simulink model "torch_pos_with_sensors_tuning(1)"  (R2024a)
settings: Solver=FixedStepAuto  StartTime=0.0  StopTime=50  FixedStep=framePeriod_s  RelTol=1e-3
undefined symbols (not defined in the file): Aircraft, DiscIntNeverNeededParam, framePeriod_s, frameRate_hz, magnitude
libraries: simulink x37, slpidlib x10, simulink_extras x2, dspmathops x1
(part 1 of 4)
settings Model: Creator=brian  LastModifiedBy=lucal
settings SolverCC: AlgebraicLoopSolver=TrustRegion
settings OptimizationCC: DefaultParameterBehavior=Inlined  GainParamInheritBuiltInType=on  UseFloatMulNetSlope=on  DefaultUnderspecifiedDataType=single  EnhancedBackFolding=on  BooleansAsBitfields=on  PassReuseOutputArgsAs=Individual arguments  StateBitsets=on  DataBitsets=on  ActiveStateOutputEnumStorageType=uint16  ZeroExternalMemoryAtStartup=off  ZeroInternalMemoryAtStartup=off  EfficientFloat2IntCast=on  LifeSpan=inf  DifferentSizesBufferReuse=on  OptimizationPriority=RAM  OptimizationCustomize=off  EfficientTunableParamExpr=on
settings DebuggingCC: ParameterPrecisionLossMsg=none  ParameterTunabilityLossMsg=error  UnconnectedInputMsg=warning  UnconnectedOutputMsg=warning  UnconnectedLineMsg=warning  BusObjectLabelMismatch=error  RootOutportRequireBusObject=error  NonBusSignalsTreatedAsBus=error  SFInvalidInputDataAccessInChartInitDiag=error  SFTransitionOutsideNaturalParentDiag=error  SFUnreachableExecutionPathDiag=error  SFUndirectedBroadcastEventsDiag=error
settings HardwareCC: ProdBitPerPointer=32  ProdBitPerSizeT=32  ProdBitPerPtrDiffT=32  ProdLargestAtomicInteger=Long  ProdLargestAtomicFloat=Double  ProdWordSize=32  ProdHWDeviceType=NXP->Cortex-M4  TargetLargestAtomicInteger=Long  TargetLargestAtomicFloat=Double  TargetLongLongMode=on  TargetIntDivRoundTo=Zero  TargetEndianess=LittleEndian  TargetHWDeviceType=NXP->Cortex-M4  ProdEqTarget=off
settings ModelReferenceCC: EnableRefExpFcnMdlSchedulingChecks=on  ModelReferenceNumInstancesAllowed=Single
settings SFSimCC: SimParseCustomCode=off  SimGenImportedTypeDefs=on  MATLABDynamicMemAlloc=off  SimTargetLang=C++
settings SFSimCC: SimUserIncludeDirs=|
  | ../../flight_code/include
  | ../../../ua_spaaro_extra/imu/include
  | ../../../ua_spaaro_extra/gnss/include
  | ../../../ua_spaaro_extra/pres/include
  | ../../../ua_spaaro_extra/sbus/include
  | ../../../ua_spaaro_extra/global_defs/include
settings SFSimCC: SimUserDefines=|
  | SIL
  | __FMU_R_MINI_V1__
settings RTWCC: Description=Embedded Coder  SystemTargetFile=ert.tlc  GenCodeOnly=on  TemplateMakefile=ert_default_tmf  GenerateReport=on  RTWVerbose=off  RTWUseSimCustomCode=on  Toolchain=MinGW64 | gmake (64-bit Windows)  BuildConfiguration=Specify  IncludeHyperlinkInReport=on  LaunchReport=on  TargetLang=C++  GenerateTraceInfo=on  GenerateTraceReport=on  GenerateTraceReportSl=on  GenerateTraceReportSf=on  GenerateTraceReportEml=on  GenerateCodeReplacementReport=on  GPUComputeCapability=3.5  DLArmComputeVersion=19.05
settings RTWCC: CustomInclude=|
  | ../../flight_code/include
  | ../../../ua_spaaro_extra/imu/include
  | ../../../ua_spaaro_extra/gnss/include
  | ../../../ua_spaaro_extra/pres/include
  | ../../../ua_spaaro_extra/sbus/include
  | ../../../ua_spaaro_extra/global_defs/include
settings RTWCC: CustomDefine=|
  | SIL
  | __FMU_R_MINI_V1__
settings CodeAppCC: ForceParamTrailComments=on  IgnoreCustomStorageClasses=off  OperatorAnnotations=on  SimulinkDataObjDesc=on  SFDataObjDesc=on  MATLABFcnDesc=on  CustomSymbolStrGlobalVar=rt$N$M  CustomSymbolStrType=$N$M  CustomSymbolStrFcn=$N$M$F  CustomSymbolStrMacro=$N$M  InsertBlockDesc=on  StateflowObjectComments=on  MATLABSourceComments=on  EnableCustomComments=on  InternalIdentifier=Classic  InlinedPrmAccess=Macros  ReqsInCode=on
settings ERTTargetCC: TargetLangStandard=C++03 (ISO)  GenerateFullHeader=off  IncludeMdlTerminateFcn=off  CombineSignalStateStructs=on  SuppressErrorStatus=on  SupportAbsoluteTime=off  CodeInterfacePackaging=C++ class  SupportNonFinite=off  SupportComplex=off  ParenthesesLevel=Standards  CastingMode=Standards  ERTHeaderFileRootName=autocode$E  ERTSourceFileRootName=autocode$E  InlinedParameterPlacement=NonHierarchical  RootIOFormat=Structure reference  ERTCustomFileTemplate=example_file_process.tlc  ERTFilePackagingFormat=Compact  PreserveExpressionOrder=on  PreserveIfCondition=on  ConvertIfToSwitch=off  EnableSignedLeftShifts=off  EnableSignedRightShifts=off  IndentSize=4

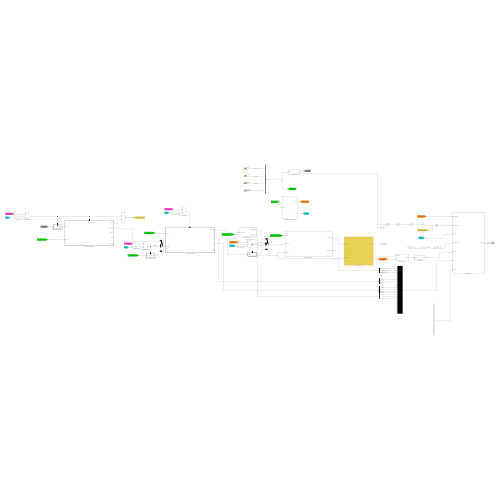
[thumbnail: Simulink's stored preview of the top-level diagram]
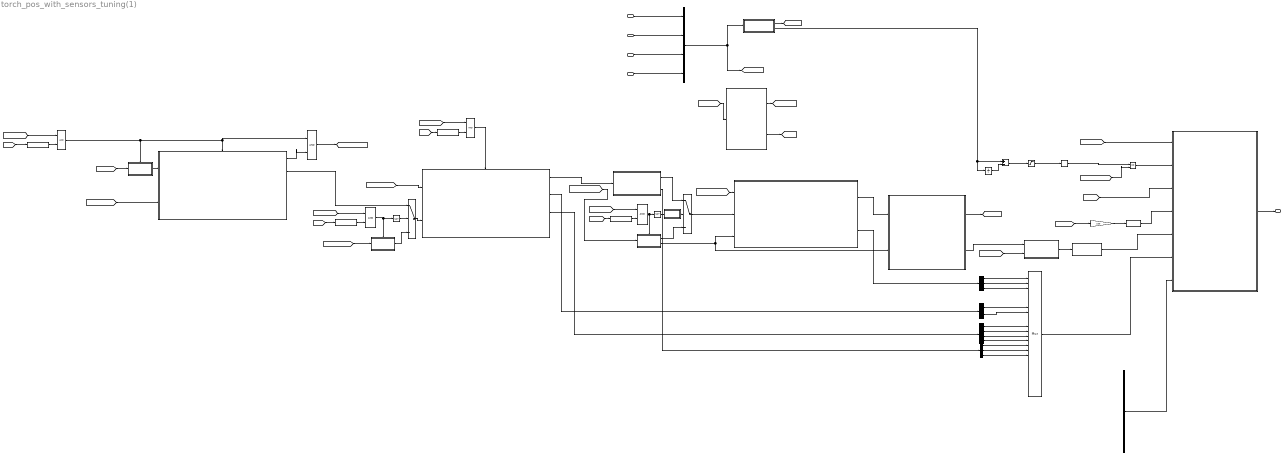
== system torch_pos_with_sensors_tuning(1) ==
  System Data : Inport  OutDataTypeStr=Bus: SysData  SampleTime=framePeriod_s  BusOutputAsStruct=on
  Sensor Data : Inport  Port=2  OutDataTypeStr=Bus: SensorData  SampleTime=framePeriod_s  BusOutputAsStruct=on
  StateEstData : Inport  Port=3  OutDataTypeStr=Bus: StateEstData  SampleTime=framePeriod_s  BusOutputAsStruct=on
  Telemetry Data : Inport  Port=4  OutDataTypeStr=Bus: TelemData  SampleTime=framePeriod_s  BusOutputAsStruct=on
  AND : Logic  IconShape=distinctive  AllPortsSameDT=off  OutDataTypeStr=boolean
  ANGLE CONTROLLER1 : Subsystem
  Bus Creator1 : BusCreator  Inputs=4
  Bus Selector : BusSelector  OutputSignals=throttle,pitch_rate_cmd,pitch_angle_cmd_rad
  Bus Selector1 : BusSelector  OutputSignals=ve_x_cmd,ve_x
  Bus Selector2 : BusSelector  OutputSignals=vz_cmd,vz,tar_z,cur_z
  Cast : DataTypeConversion  OutDataTypeStr=single  SaturateOnIntegerOverflow=off  RndMeth=Floor
  Compare To Constant : simulink/Logic and Bit Operations/Compare To Constant  relop=>  const=0.5  OutDataTypeStr=boolean
  Demux : Demux  Outputs=3
  Gain : Gain  Gain=100
  Motor Mixing Algorithm : Subsystem
  Mux : Mux  Inputs=24
  Mux1 : Mux  Inputs=16
  NOT : Logic  Operator=NOT  IconShape=distinctive  AllPortsSameDT=off  OutDataTypeStr=boolean
  NOT1 : Logic  Operator=NOT  IconShape=distinctive  AllPortsSameDT=off  OutDataTypeStr=boolean
  OR : Logic  Operator=OR  IconShape=distinctive  AllPortsSameDT=off  OutDataTypeStr=boolean
  OUTER_TO_INNER_CONV : Subsystem
  POS_HOLD CONTROLLER : Subsystem
  POS_HOLD_input_conversion : Subsystem
  Saturation : Saturate  UpperLimit=1  LowerLimit=0
  Stab_input_conversion : Subsystem
  Subtract : Sum  Inputs=+-
  Switch : Switch  Criteria=u2 > Threshold  Threshold=0.5  SaturateOnIntegerOverflow=off  InputSameDT=off
  Switch1 : Switch  Criteria=u2 > Threshold  Threshold=0.5  SaturateOnIntegerOverflow=off  InputSameDT=off
  To VMS Data : Subsystem
  Unit Delay : UnitDelay  SampleTime=-1  HasFrameUpgradeWarning=on
  WAYPOINT CONTROLLER : Subsystem
  WAYPOINT CONTROLLER CMD : Subsystem
  cmd to raw pwm1 : Subsystem
  command selection : Subsystem
  compare_to_pos_hold : simulink/Logic and Bit Operations/Compare To Constant  relop=>=  const=2  OutDataTypeStr=boolean
  compare_to_stab : simulink/Logic and Bit Operations/Compare To Constant  relop===  const=1  OutDataTypeStr=boolean
  compare_to_stab1 : simulink/Logic and Bit Operations/Compare To Constant  relop===  const=2  OutDataTypeStr=boolean
  compare_to_wp : simulink/Logic and Bit Operations/Compare To Constant  relop=>=  const=3  OutDataTypeStr=boolean
  delayed : Subsystem
  determine arm and mode selection : Subsystem
  emergency_stop_system1 : Subsystem
  motor_armed AND mode 2 : Logic  IconShape=distinctive  AllPortsSameDT=off  OutDataTypeStr=boolean
  motor_armed AND mode_0 : Logic  IconShape=distinctive  AllPortsSameDT=off  OutDataTypeStr=boolean
  motor_armed AND mode_1 : Logic  IconShape=distinctive  AllPortsSameDT=off  OutDataTypeStr=boolean
  motor_armed AND mode_2 : Logic  IconShape=distinctive  AllPortsSameDT=off  OutDataTypeStr=boolean
  VmsData : Outport  OutDataTypeStr=Bus: VmsData  SampleTime=framePeriod_s  BusOutputAsStruct=on
  wires:
  To VMS Data/1(VmsData) -> VmsData/1  "VmsData"
  [Mode] -> To VMS Data/3(Mode in)
  [arm_state] -> To VMS Data/1(motors_enabled)
  Cast/1 -> To VMS Data/4(throttle_cmd_prcnt)
  [throttle] -> Gain/1
  Gain/1 -> Cast/1
  command selection/1(cmd) -> [cmd]
  Bus Creator1/1 -> command selection/1(InBus), [sys_input]
  [sys_input] -> determine arm and mode selection/1(sys_input)
  Motor Mixing Algorithm/2(PWM) -> emergency_stop_system1/1(input_signal)
  cmd to raw pwm1/1(PwmCmd) -> To VMS Data/5(PWM In)  "PwmCmd"
  emergency_stop_system1/1(pwm_cmd) -> cmd to raw pwm1/1(pwm_cmd)
  Mux/1 -> To VMS Data/6(Aux)
  [arm_state] -> emergency_stop_system1/2(arm)
  compare_to_stab/1 -> motor_armed AND mode_0/2
  [sys_input] -> ANGLE CONTROLLER1/1(Sys_input)
  [arm_state] -> motor_armed AND mode_0/1
  motor_armed AND mode_0/1 -> Stab_input_conversion/Enable, NOT/1
  Stab_input_conversion/1(angle_ctrl_input) -> Switch/3
  [Mode] -> compare_to_stab/1
  ANGLE CONTROLLER1/1(Command out) -> Motor Mixing Algorithm/1(MMA Bus)
  compare_to_pos_hold/1 -> motor_armed AND mode_1/2
  motor_armed AND mode 2/1 -> NOT1/1, POS_HOLD_input_conversion/Enable
  [Mode] -> compare_to_pos_hold/1
  [arm_state] -> motor_armed AND mode_1/1
  NOT1/1 -> Switch1/2
  [arm_state] -> motor_armed AND mode 2/1
  [Mode] -> compare_to_stab1/1
  motor_armed AND mode_1/1 -> POS_HOLD CONTROLLER/Enable
  compare_to_stab1/1 -> motor_armed AND mode 2/2
  Stab_input_conversion/2(low_throttle) -> ANGLE CONTROLLER1/3(low_thottle), Motor Mixing Algorithm/2(low_throttle_flag)
  System Data/1 -> Bus Creator1/1  "Sys Data"
  Sensor Data/1 -> Bus Creator1/2  "Sensor Data"
  StateEstData/1 -> Bus Creator1/3  "StateEstData"
  [sys_input] -> POS_HOLD CONTROLLER/1(Sys_input)
  AND/1 -> [waypoint_reached]
  motor_armed AND mode_2/1 -> WAYPOINT CONTROLLER CMD/Enable, WAYPOINT CONTROLLER/Enable, AND/1
  [arm_state] -> motor_armed AND mode_2/1
  [Mode] -> compare_to_wp/1
  compare_to_wp/1 -> motor_armed AND mode_2/2
  [cmd] -> WAYPOINT CONTROLLER CMD/1(cmd)
  POS_HOLD_input_conversion/1(angle_ctrl_input) -> Switch1/3
  Switch1/1 -> POS_HOLD CONTROLLER/2(param_input)
  POS_HOLD CONTROLLER/2(Output) -> Bus Selector1/1
  WAYPOINT CONTROLLER CMD/1(angle_ctrl_input) -> WAYPOINT CONTROLLER/1(cmd)
  [sys_input] -> WAYPOINT CONTROLLER/2(Sys_input)
  WAYPOINT CONTROLLER/1(wp_reached) -> AND/2
  Mux1/1 -> To VMS Data/7(SBUS in)
  ANGLE CONTROLLER1/2(stab_mode_dbg) -> Bus Selector/1
  Bus Selector/1 -> Mux/1  "<throttle>"
  Bus Selector/2 -> Mux/2  "<pitch_rate_cmd>"
  Bus Selector/3 -> Mux/3  "<pitch_angle_cmd_rad>"
  Bus Selector1/1 -> Mux/7  "<ve_x_cmd>"
  Bus Selector1/2 -> Mux/8  "<ve_x>"
  command selection/2(skip_wp) -> Unit Delay/1, Subtract/1
  Unit Delay/1 -> Subtract/2
  Subtract/1 -> Saturation/1
  Saturation/1 -> Compare To Constant/1
  Telemetry Data/1 -> Bus Creator1/4  "Telemetry Data"
  [sys_input] -> Stab_input_conversion/1(sys_input)
  Switch/1 -> ANGLE CONTROLLER1/2(Param_input)
  Motor Mixing Algorithm/1(throttle) -> [throttle]
  delayed/1(delayed_sig) -> Switch/2
  NOT/1 -> delayed/1(sig)
  POS_HOLD CONTROLLER/1(Command out) -> OUTER_TO_INNER_CONV/1(Outer loop command)
  OUTER_TO_INNER_CONV/1(Inner loop command) -> Switch/1
  WAYPOINT CONTROLLER/2(wp_command) -> Switch1/1
  [sys_input] -> POS_HOLD_input_conversion/1(Sys)
  OR/1 -> To VMS Data/2(waypoint_reached)
  Compare To Constant/1 -> OR/1
  [waypoint_reached] -> OR/2
  POS_HOLD CONTROLLER/3(Output1) -> Bus Selector2/1
  Bus Selector2/1 -> Mux/11  "<vz_cmd>"
  Bus Selector2/2 -> Mux/12  "<vz>"
  Bus Selector2/3 -> Mux/13  "<tar_z>"
  Bus Selector2/4 -> Mux/14  "<cur_z>"
  OUTER_TO_INNER_CONV/2(thrust_vector_cmd) -> Demux/1
  Demux/3 -> Mux/17
  Demux/2 -> Mux/16
  Demux/1 -> Mux/15
  determine arm and mode selection/1(arm_state) -> [arm_state]
  determine arm and mode selection/2(mode) -> [Mode]

== system torch_pos_with_sensors_tuning(1)/ANGLE CONTROLLER1 ==
  Sys_input : Inport
  Param_input : Inport  Port=2
  low_thottle : Inport  Port=3
  Bus Creator : BusCreator  Inputs=3
  Bus Creator4 : BusCreator  Inputs=4
  Bus Selector : BusSelector  OutputSignals=throttle_cc,pitch_angle_cmd_rad
  Ground : Ground
  Ground2 : Ground
  Pitch Controller : Subsystem
  Command out : Outport
  stab_mode_dbg : Outport  Port=2
  wires:
  Bus Creator4/1 -> Command out/1
  Param_input/1 -> Bus Selector/1
  Ground2/1 -> Bus Creator4/4  "yaw_cc"
  Pitch Controller/1(pitch_cc) -> Bus Creator4/3  "pitch_cc"
  Ground/1 -> Bus Creator4/2  "roll_cc"
  Sys_input/1 -> Pitch Controller/1(sys_input)
  Bus Selector/1 -> [throttle_cc]  "<throttle_cc>"
  Bus Selector/2 -> [pitch_angle_cmd_rad]  "<pitch_angle_cmd_rad>"
  [throttle_cc] -> Bus Creator/1, Bus Creator4/1  "throttle"
  [pitch_angle_cmd_rad] -> Pitch Controller/2(Pitch_angle_cmd)
  low_thottle/1 -> [low_throttle_flag]
  [low_throttle_flag] -> Pitch Controller/3(low_throttle_flag)
  Bus Creator/1 -> stab_mode_dbg/1
  [pitch_angle_cmd_rad] -> Bus Creator/3
  Pitch Controller/2(pitch_rate_cmd) -> Bus Creator/2

== system torch_pos_with_sensors_tuning(1)/Motor Mixing Algorithm ==
  MMA Bus : Inport
  low_throttle_flag : Inport  Port=2
  Bus Selector : BusSelector  OutputSignals=throttle,roll_cc,pitch_cc,yaw_cc
  Constant : Constant  OutDataTypeStr=single
  Constant1 : Constant  Value=Aircraft.Control.motor_spin_min  OutDataTypeStr=single
  Constant2 : Constant  Value=[0 0 0 0 0 0 0 0]  OutDataTypeStr=single
  Motor Mix : Constant  Value=Aircraft.Motor.mix  OutDataTypeStr=single
  Multiply : Product  Inputs=**  Multiplication=Matrix(*)  OutDataTypeStr=single
  Mux : Mux
  Reshape : Reshape  OutputDimensionality=Row vector (2-D)
  Saturation Dynamic : simulink/Discontinuities/Saturation Dynamic  OutMin=[]  OutMax=[]  OutDataTypeStr=Inherit: Same as second input  OutDataType=fixdt(1, 16)  OutScaling=2^-10  DoSatur=off
  Switch : Switch  Criteria=u2 > Threshold  SaturateOnIntegerOverflow=off  InputSameDT=off
  Transpose : Math  Operator=transpose
  throttle : Outport
  PWM : Outport  Port=2
  wires:
  Mux/1 -> Reshape/1
  Reshape/1 -> Multiply/1
  Motor Mix/1 -> Transpose/1
  MMA Bus/1 -> Bus Selector/1
  Bus Selector/1 -> Mux/1, throttle/1  "<throttle>"
  Transpose/1 -> Multiply/2
  Saturation Dynamic/1 -> PWM/1
  Constant/1 -> Saturation Dynamic/1
  Constant1/1 -> Saturation Dynamic/3
  Bus Selector/2 -> Mux/2  "<roll_cc>"
  Bus Selector/3 -> Mux/3  "<pitch_cc>"
  Bus Selector/4 -> Mux/4  "<yaw_cc>"
  Switch/1 -> Saturation Dynamic/2
  low_throttle_flag/1 -> Switch/2
  Multiply/1 -> Switch/3  "Command"
  Constant2/1 -> Switch/1

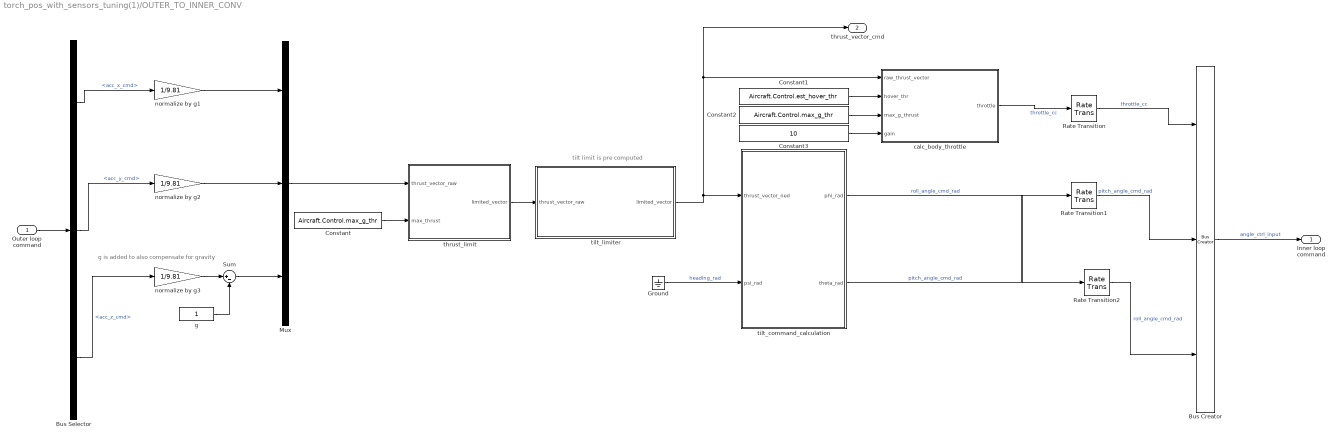
== system torch_pos_with_sensors_tuning(1)/OUTER_TO_INNER_CONV ==
  note: g is added to also compensate for gravity
  note: tilt limit is pre computed
  Outer loop command : Inport
  " tilt_limiter" : MATLAB Function  TreatAsAtomicUnit=on
  Bus Creator : BusCreator  Inputs=3
  Bus Selector : BusSelector  OutputSignals=acc_x_cmd,acc_y_cmd,acc_z_cmd
  Constant : Constant  Value=Aircraft.Control.max_g_thr  OutDataTypeStr=single
  Constant1 : Constant  Value=Aircraft.Control.est_hover_thr  OutDataTypeStr=single
  Constant2 : Constant  Value=Aircraft.Control.max_g_thr  OutDataTypeStr=single
  Constant3 : Constant  Value=10  OutDataTypeStr=single
  Ground : Ground
  Mux : Mux  Inputs=3
  Rate Transition : RateTransition  OutPortSampleTime=0.01
  Rate Transition1 : RateTransition  OutPortSampleTime=0.01
  Rate Transition2 : RateTransition  OutPortSampleTime=0.01
  Sum : Sum  Inputs=|+-
  calc_body_throttle : MATLAB Function  TreatAsAtomicUnit=on
  g : Constant  OutDataTypeStr=single
  normalize by g1 : Gain  Gain=1/9.81
  normalize by g2 : Gain  Gain=1/9.81
  normalize by g3 : Gain  Gain=1/9.81
  thrust_limit : MATLAB Function  TreatAsAtomicUnit=on
  tilt_command_calculation : MATLAB Function  TreatAsAtomicUnit=on
  Inner loop command : Outport
  thrust_vector_cmd : Outport  Port=2
  wires:
  Constant/1 -> thrust_limit/2(max_thrust)
  Mux/1 -> thrust_limit/1(thrust_vector_raw)
  Outer loop command/1 -> Bus Selector/1
  Bus Selector/1 -> normalize by g1/1  "<acc_x_cmd>"
  Bus Selector/2 -> normalize by g2/1  "<acc_y_cmd>"
  Bus Creator/1 -> Inner loop command/1  "angle_ctrl_input"
  Ground/1 -> tilt_command_calculation/2(psi_rad)  "heading_rad"
  Bus Selector/3 -> normalize by g3/1  "<acc_z_cmd>"
  g/1 -> Sum/2
  normalize by g3/1 -> Sum/1
  normalize by g1/1 -> Mux/1
  normalize by g2/1 -> Mux/2
  Sum/1 -> Mux/3
  thrust_limit/1(limited_vector) -> " tilt_limiter"/1(thrust_vector_raw)
  tilt_command_calculation/1(phi_rad) -> Rate Transition2/1  "roll_angle_cmd_rad"
  tilt_command_calculation/2(theta_rad) -> Rate Transition1/1  "pitch_angle_cmd_rad"
  calc_body_throttle/1(throttle) -> Rate Transition/1  "throttle_cc"
  " tilt_limiter"/1(limited_vector) -> tilt_command_calculation/1(thrust_vector_ned), thrust_vector_cmd/1, calc_body_throttle/1(raw_thrust_vector)
  Constant1/1 -> calc_body_throttle/2(hover_thr)
  Constant2/1 -> calc_body_throttle/3(max_g_thrust)
  Constant3/1 -> calc_body_throttle/4(gain)
  Rate Transition/1 -> Bus Creator/1  "throttle_cc"
  Rate Transition1/1 -> Bus Creator/2  "pitch_angle_cmd_rad"
  Rate Transition2/1 -> Bus Creator/3  "roll_angle_cmd_rad"

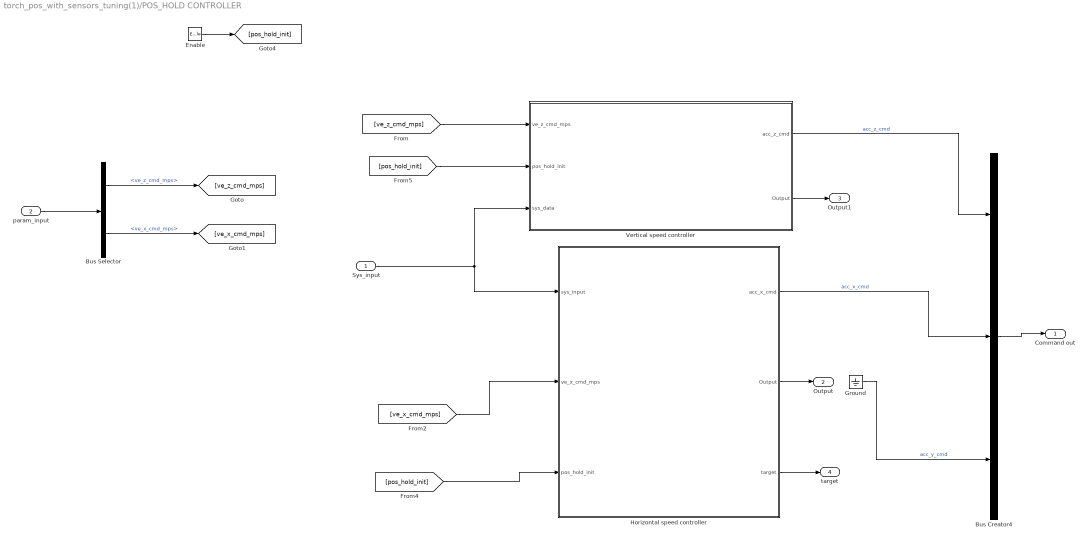
== system torch_pos_with_sensors_tuning(1)/POS_HOLD CONTROLLER ==
  Sys_input : Inport
  param_input : Inport  Port=2
  Enable : EnablePort  StatesWhenEnabling=reset  PropagateVarSize=During execution  ShowOutputPort=on
  Bus Creator4 : BusCreator  Inputs=3
  Bus Selector : BusSelector  OutputSignals=ve_z_cmd_mps,ve_x_cmd_mps
  Ground : Ground
  Horizontal speed controller : Subsystem
  Vertical speed controller : Subsystem
  Command out : Outport
  Output : Outport  Port=2
  Output1 : Outport  Port=3
  target : Outport  Port=4
  wires:
  Bus Creator4/1 -> Command out/1
  Bus Selector/1 -> [ve_z_cmd_mps]  "<ve_z_cmd_mps>"
  Bus Selector/2 -> [ve_x_cmd_mps]  "<ve_x_cmd_mps>"
  param_input/1 -> Bus Selector/1
  Enable/1 -> [pos_hold_init]
  Vertical speed controller/1(acc_z_cmd) -> Bus Creator4/1  "acc_z_cmd"
  Horizontal speed controller/1(acc_x_cmd) -> Bus Creator4/2  "acc_x_cmd"
  Ground/1 -> Bus Creator4/3  "acc_y_cmd"
  [ve_x_cmd_mps] -> Horizontal speed controller/2(ve_x_cmd_mps)
  Sys_input/1 -> Vertical speed controller/3(sys_data), Horizontal speed controller/1(sys_input)
  [pos_hold_init] -> Horizontal speed controller/3(pos_hold_init)
  Horizontal speed controller/2(Output) -> Output/1
  [ve_z_cmd_mps] -> Vertical speed controller/1(ve_z_cmd_mps)
  [pos_hold_init] -> Vertical speed controller/2(pos_hold_init)
  Vertical speed controller/2(Output) -> Output1/1
  Horizontal speed controller/3(target) -> target/1

== system torch_pos_with_sensors_tuning(1)/POS_HOLD_input_conversion ==
  Sys : Inport
  Enable : EnablePort
  Bus Creator : BusCreator  Inputs=4
  Bus Selector2 : BusSelector  OutputSignals=Telemetry Data.param
  Cast1 : DataTypeConversion  OutDataTypeStr=single  SaturateOnIntegerOverflow=off  RndMeth=Floor
  Cast2 : DataTypeConversion  OutDataTypeStr=single  SaturateOnIntegerOverflow=off  RndMeth=Floor
  Constant3 : Constant  Value=-0.5
  Constant4 : Constant  Value=0.5
  Constant5 : Constant  Value=-0.5
  Constant6 : Constant  Value=0.5
  Ground : Ground
  Ground2 : Ground
  Saturation Dynamic : simulink/Discontinuities/Saturation Dynamic  OutMin=[]  OutMax=[]  OutDataTypeStr=double  OutDataType=fixdt(1, 16)  OutScaling=2^-10  DoSatur=off
  Saturation Dynamic1 : simulink/Discontinuities/Saturation Dynamic  OutMin=[]  OutMax=[]  OutDataTypeStr=double  OutDataType=fixdt(1, 16)  OutScaling=2^-10  DoSatur=off
  Selector : Selector  IndexMode=Zero-based  InputPortWidth=24  IndexOptions=Index vector (dialog)  Indices=1  OutputSizes=1
  Selector1 : Selector  IndexMode=Zero-based  InputPortWidth=24  IndexOptions=Index vector (dialog)  Indices=2  OutputSizes=1
  angle_ctrl_input : Outport
  wires:
  Bus Creator/1 -> angle_ctrl_input/1  "pos_hold_cmd"
  Saturation Dynamic/1 -> Bus Creator/1  "ve_z_cmd_mps"
  Saturation Dynamic1/1 -> Bus Creator/2  "ve_x_cmd_mps"
  Ground2/1 -> Bus Creator/3  "ve_y_cmd_mps"
  Sys/1 -> Bus Selector2/1
  Constant5/1 -> Saturation Dynamic/3
  Constant6/1 -> Saturation Dynamic/1
  Cast1/1 -> Saturation Dynamic/2
  Selector/1 -> Cast1/1
  Bus Selector2/1 -> Selector1/1, Selector/1  "<param>"
  Ground/1 -> Bus Creator/4  "yaw_rate_cmd_radps"
  Constant4/1 -> Saturation Dynamic1/1
  Constant3/1 -> Saturation Dynamic1/3
  Cast2/1 -> Saturation Dynamic1/2
  Selector1/1 -> Cast2/1

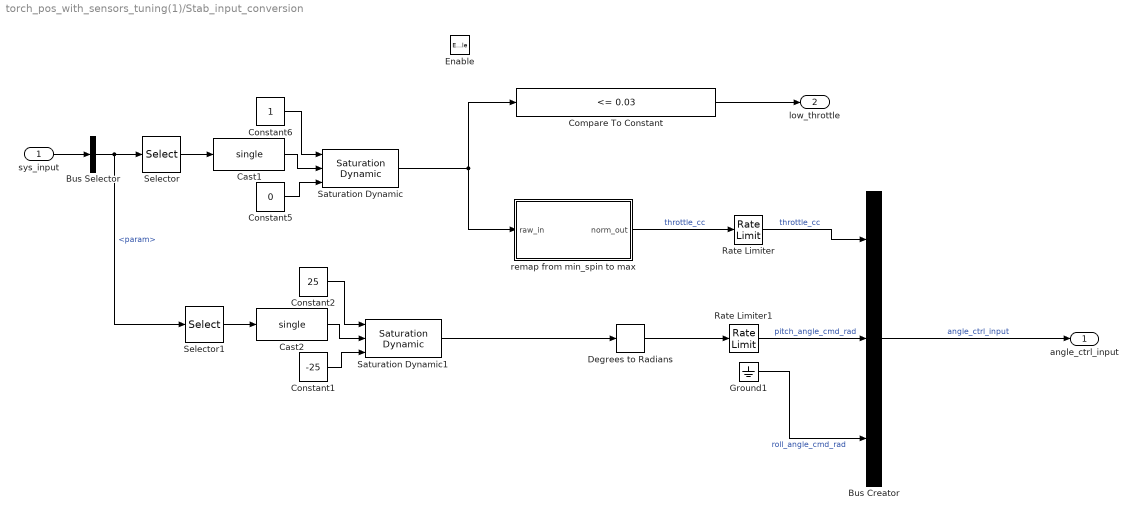
== system torch_pos_with_sensors_tuning(1)/Stab_input_conversion ==
  sys_input : Inport
  Enable : EnablePort
  Bus Creator : BusCreator  Inputs=3
  Bus Selector : BusSelector  OutputSignals=Telemetry Data.param
  Cast1 : DataTypeConversion  OutDataTypeStr=single  SaturateOnIntegerOverflow=off  RndMeth=Floor
  Cast2 : DataTypeConversion  OutDataTypeStr=single  SaturateOnIntegerOverflow=off  RndMeth=Floor
  Compare To Constant : simulink/Logic and Bit Operations/Compare To Constant  relop=<=  const=0.03  OutDataTypeStr=boolean
  Constant1 : Constant  Value=-25
  Constant2 : Constant  Value=25
  Constant5 : Constant  Value=0
  Constant6 : Constant
  Degrees to Radians : simulink_extras/Transformations/Degrees to Radians
  Ground1 : Ground
  Rate Limiter : RateLimiter  SampleTimeMode=inherited
  Rate Limiter1 : RateLimiter  RisingSlewLimit=2  SampleTimeMode=inherited
  Saturation Dynamic : simulink/Discontinuities/Saturation Dynamic  OutMin=[]  OutMax=[]  OutDataTypeStr=double  OutDataType=fixdt(1, 16)  OutScaling=2^-10  DoSatur=off
  Saturation Dynamic1 : simulink/Discontinuities/Saturation Dynamic  OutMin=[]  OutMax=[]  OutDataTypeStr=double  OutDataType=fixdt(1, 16)  OutScaling=2^-10  DoSatur=off
  Selector : Selector  IndexMode=Zero-based  InputPortWidth=24  IndexOptions=Index vector (dialog)  Indices=1  OutputSizes=1
  Selector1 : Selector  IndexMode=Zero-based  InputPortWidth=24  IndexOptions=Index vector (dialog)  Indices=2  OutputSizes=1
  remap from min_spin to max : Subsystem
  angle_ctrl_input : Outport
  low_throttle : Outport  Port=2
  wires:
  Ground1/1 -> Bus Creator/3  "roll_angle_cmd_rad"
  remap from min_spin to max/1(norm_out) -> Rate Limiter/1  "throttle_cc"
  Bus Creator/1 -> angle_ctrl_input/1  "angle_ctrl_input"
  Saturation Dynamic1/1 -> Degrees to Radians/1
  sys_input/1 -> Bus Selector/1
  Constant5/1 -> Saturation Dynamic/3
  Constant6/1 -> Saturation Dynamic/1
  Bus Selector/1 -> Selector1/1, Selector/1  "<param>"
  Selector/1 -> Cast1/1
  Cast1/1 -> Saturation Dynamic/2
  Compare To Constant/1 -> low_throttle/1
  Saturation Dynamic/1 -> Compare To Constant/1, remap from min_spin to max/1(raw_in)
  Rate Limiter/1 -> Bus Creator/1  "throttle_cc"
  Constant1/1 -> Saturation Dynamic1/3
  Selector1/1 -> Cast2/1
  Cast2/1 -> Saturation Dynamic1/2
  Constant2/1 -> Saturation Dynamic1/1
  Degrees to Radians/1 -> Rate Limiter1/1
  Rate Limiter1/1 -> Bus Creator/2  "pitch_angle_cmd_rad"

== system torch_pos_with_sensors_tuning(1)/To VMS Data ==
  motors_enabled : Inport
  waypoint_reached : Inport  Port=2
  Mode in : Inport  Port=3
  throttle_cmd_prcnt : Inport  Port=4
  PWM In : Inport  Port=5
  Aux : Inport  Port=6
  SBUS in : Inport  Port=7
  Bus Creator : BusCreator  Inputs=9  OutDataTypeStr=Bus: VmsData  NonVirtualBus=on
      settings: InheritFromInputs=off
  Ground : Ground
  Ground2 : Ground
  VmsData : Outport
  wires:
  Bus Creator/1 -> VmsData/1
  waypoint_reached/1 -> Bus Creator/1  "advance_waypoint"
  motors_enabled/1 -> Bus Creator/2  "motors_enabled"
  Mode in/1 -> Bus Creator/3  "mode"
  SBUS in/1 -> Bus Creator/4  "sbus"
  PWM In/1 -> Bus Creator/5  "pwm"
  throttle_cmd_prcnt/1 -> Bus Creator/6  "throttle_cmd_prcnt"
  Aux/1 -> Bus Creator/9  "aux"
  Ground/1 -> Bus Creator/7  "flight_time_remaining_s"
  Ground2/1 -> Bus Creator/8  "power_remaining_prcnt"

== system torch_pos_with_sensors_tuning(1)/WAYPOINT CONTROLLER ==
  cmd : Inport
  Sys_input : Inport  Port=2
  Enable : EnablePort  StatesWhenEnabling=reset  ShowOutputPort=on
  Bus Selector1 : BusSelector  OutputSignals=Telemetry Data.waypoints_updated,Telemetry Data.current_waypoint
  Constant : Constant  OutDataTypeStr=int16
  OR : Logic  Operator=OR  Inputs=3  IconShape=distinctive  AllPortsSameDT=off  OutDataTypeStr=boolean
  Sum : Sum  Inputs=|++
  Unit Delay : UnitDelay  SampleTime=-1  HasFrameUpgradeWarning=on
  WP_NAV : Subsystem
  capture rising edge : Subsystem
  determine target : Subsystem
  wp_completion_check : Subsystem
  wp_reached : Outport
  wp_command : Outport  Port=2
  tar_pos_m : Outport  Port=3
  cur_wp : Outport  Port=4
  bearing_to_tar : Outport  Port=5
  wires:
  Sys_input/1 -> Bus Selector1/1, WP_NAV/2(Sys_input), wp_completion_check/2(Sys_input), determine target/1(sys_input)
  Enable/1 -> WP_NAV/Enable
  WP_NAV/1(Command out) -> wp_command/1
  determine target/1(cur_target_pos_m) -> wp_completion_check/1(target_pos), tar_pos_m/1, WP_NAV/3(cur_target_pos_m)  "cur_target_pos_m"
  OR/1 -> determine target/Enable  "enable"
  Bus Selector1/1 -> OR/1  "<waypoints_updated>"
  capture rising edge/1(enable) -> OR/2
  Unit Delay/1 -> OR/3
  cmd/1 -> WP_NAV/1(Cmd)
  wp_completion_check/1(wp_reached) -> wp_reached/1, Unit Delay/1
  Constant/1 -> Sum/2
  Bus Selector1/2 -> Sum/1  "<current_waypoint>"
  Sum/1 -> cur_wp/1, capture rising edge/1(<current_waypoint>)  "cur_wp"
  determine target/2(prev_pos_m) -> WP_NAV/4(prev_pos_m)  "prev_wp"
  determine target/3(max_v_xy_mps) -> WP_NAV/5(max_v_hor_mps)
  determine target/4(max_v_z_mps) -> WP_NAV/6(max_v_z_mps)
  WP_NAV/2(nav_data) -> bearing_to_tar/1

== system torch_pos_with_sensors_tuning(1)/WAYPOINT CONTROLLER CMD ==
  cmd : Inport
  Enable : EnablePort
  Bus Creator : BusCreator  Inputs=4
  Bus Selector2 : BusSelector  OutputSignals=throttle,pitch,roll,yaw
  Constant : Constant  Commented=on  Value=Aircraft.Inceptor.deadband
  Constant1 : Constant  Value=Aircraft.Control.v_hor_max  OutDataTypeStr=single
  Constant4 : Constant  Value=Aircraft.Control.v_hor_max  OutDataTypeStr=single
  Ground : Ground
  Product : Product
  Product1 : Product
  Product2 : Product
  Throttle Mapper : Subsystem  Commented=on
  pitch_norm_deadband : Subsystem  Commented=on
  remap from min_spin to max : Subsystem
  angle_ctrl_input : Outport
  wires:
  Bus Selector2/3 -> Product2/1  "<roll>"
  Product2/1 -> Bus Creator/3  "vb_y_cmd_mps"
  Bus Selector2/2 -> Product1/1  "<pitch>"
  Bus Creator/1 -> angle_ctrl_input/1  "angle_ctrl_input"
  Product1/1 -> Bus Creator/2  "vb_x_cmd_mps"
  cmd/1 -> Bus Selector2/1
  Product/1 -> Bus Creator/4  "yaw_rate_cmd_radps"
  Bus Selector2/4 -> Product/1  "<yaw>"
  pitch_norm_deadband/1(normalized_out) -> Throttle Mapper/1(Throttle)
  Constant/1 -> pitch_norm_deadband/2(deadband)
  Constant1/1 -> Product1/2
  Constant4/1 -> Product2/2
  Ground/1 -> Product/2
  remap from min_spin to max/1(norm_out) -> Bus Creator/1  "ve_z_cmd_mps"
  Bus Selector2/1 -> remap from min_spin to max/1(raw_in)  "<throttle>"

== system torch_pos_with_sensors_tuning(1)/cmd to raw pwm1 ==
  note: cnt - pwm output to actual hardware
  pwm_cmd : Inport
  Data Type Conversion : DataTypeConversion  OutDataTypeStr=int16  SaturateOnIntegerOverflow=off  RndMeth=Floor
  motor_PWM_denormalize : Subsystem
  PwmCmd : Outport
  wires:
  pwm_cmd/1 -> motor_PWM_denormalize/1(normalized_input)  "cmd"
  Data Type Conversion/1 -> PwmCmd/1  "cnt"
  motor_PWM_denormalize/1(raw_output) -> Data Type Conversion/1

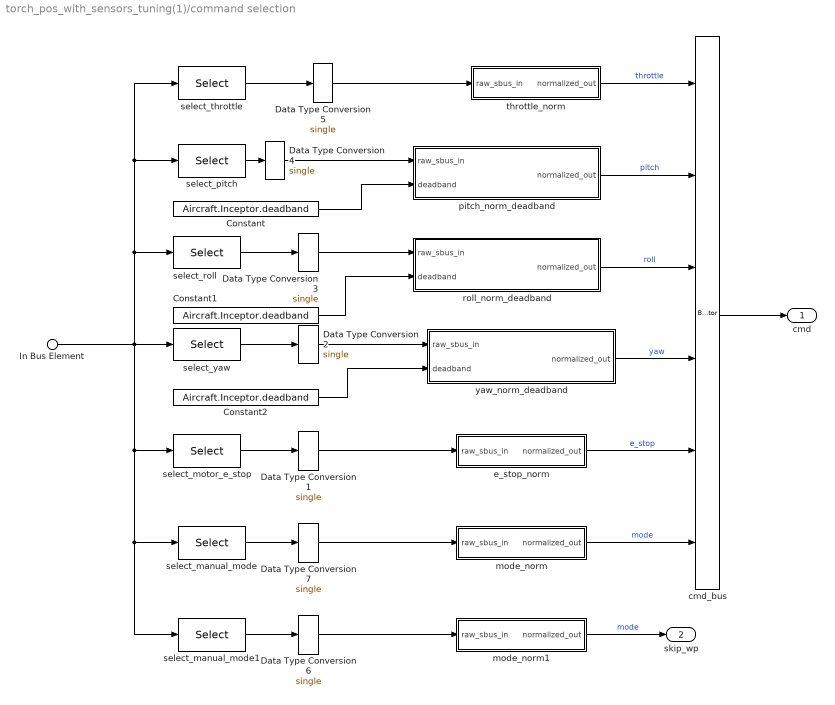
== system torch_pos_with_sensors_tuning(1)/command selection ==
  In Bus Element : Inport  PortName=InBus  Element=Sensor Data.inceptor.ch
  Constant : Constant  Value=Aircraft.Inceptor.deadband  OutDataTypeStr=single
  Constant1 : Constant  Value=Aircraft.Inceptor.deadband  OutDataTypeStr=single
  Constant2 : Constant  Value=Aircraft.Inceptor.deadband  OutDataTypeStr=single
  Data Type Conversion{1..7} (7 alike) : DataTypeConversion  OutDataTypeStr=single  SaturateOnIntegerOverflow=off  RndMeth=Floor
  cmd_bus : BusCreator  Inputs=6
  e_stop_norm : Subsystem
  mode_norm : Subsystem
  mode_norm1 : Subsystem
  pitch_norm_deadband : Subsystem
  roll_norm_deadband : Subsystem
  select_manual_mode : Selector  IndexOptions=Index vector (dialog)  Indices=Aircraft.Inceptor.mode0  OutputSizes=1
  select_manual_mode1 : Selector  IndexOptions=Index vector (dialog)  Indices=9  OutputSizes=1
  select_motor_e_stop : Selector  IndexOptions=Index vector (dialog)  Indices=Aircraft.Inceptor.throttle_e_stop  OutputSizes=1
  select_pitch : Selector  IndexOptions=Index vector (dialog)  Indices=Aircraft.Inceptor.pitch  OutputSizes=1
  select_roll : Selector  IndexOptions=Index vector (dialog)  Indices=Aircraft.Inceptor.roll  OutputSizes=1
  select_throttle : Selector  IndexOptions=Index vector (dialog)  Indices=Aircraft.Inceptor.throttle  OutputSizes=1
  select_yaw : Selector  IndexOptions=Index vector (dialog)  Indices=Aircraft.Inceptor.yaw  OutputSizes=1
  throttle_norm : Subsystem
  yaw_norm_deadband : Subsystem
  cmd : Outport
  skip_wp : Outport  Port=2
  wires:
  select_pitch/1 -> Data Type Conversion4/1
  select_yaw/1 -> Data Type Conversion2/1
  select_throttle/1 -> Data Type Conversion5/1
  cmd_bus/1 -> cmd/1
  Data Type Conversion5/1 -> throttle_norm/1(raw_sbus_in)
  select_roll/1 -> Data Type Conversion3/1
  In Bus Element/1 -> select_roll/1, select_throttle/1, select_pitch/1, select_manual_mode/1, select_manual_mode1/1, select_motor_e_stop/1, select_yaw/1
  Data Type Conversion1/1 -> e_stop_norm/1(raw_sbus_in)
  select_motor_e_stop/1 -> Data Type Conversion1/1
  Data Type Conversion7/1 -> mode_norm/1(raw_sbus_in)
  select_manual_mode/1 -> Data Type Conversion7/1
  Data Type Conversion2/1 -> yaw_norm_deadband/1(raw_sbus_in)
  Constant2/1 -> yaw_norm_deadband/2(deadband)
  throttle_norm/1(normalized_out) -> cmd_bus/1  "throttle"
  roll_norm_deadband/1(normalized_out) -> cmd_bus/3  "roll"
  pitch_norm_deadband/1(normalized_out) -> cmd_bus/2  "pitch"
  Data Type Conversion4/1 -> pitch_norm_deadband/1(raw_sbus_in)
  Constant/1 -> pitch_norm_deadband/2(deadband)
  Constant1/1 -> roll_norm_deadband/2(deadband)
  Data Type Conversion3/1 -> roll_norm_deadband/1(raw_sbus_in)
  yaw_norm_deadband/1(normalized_out) -> cmd_bus/4  "yaw"
  e_stop_norm/1(normalized_out) -> cmd_bus/5  "e_stop"
  mode_norm/1(normalized_out) -> cmd_bus/6  "mode"
  select_manual_mode1/1 -> Data Type Conversion6/1
  Data Type Conversion6/1 -> mode_norm1/1(raw_sbus_in)
  mode_norm1/1(normalized_out) -> skip_wp/1  "mode"

== system torch_pos_with_sensors_tuning(1)/delayed ==
  sig : Inport
  Constant : Constant  Value=framePeriod_s  OutDataTypeStr=single
  Constant1 : Constant  Value=0.5  OutDataTypeStr=single
  Delay : Delay  DelayLengthSource=Input port
      settings: InputPortMap=u0,p1
  Divide : Product  Inputs=*/
  delayed_sig : Outport
  wires:
  Delay/1 -> delayed_sig/1
  sig/1 -> Delay/1
  Divide/1 -> Delay/2
  Constant/1 -> Divide/2
  Constant1/1 -> Divide/1

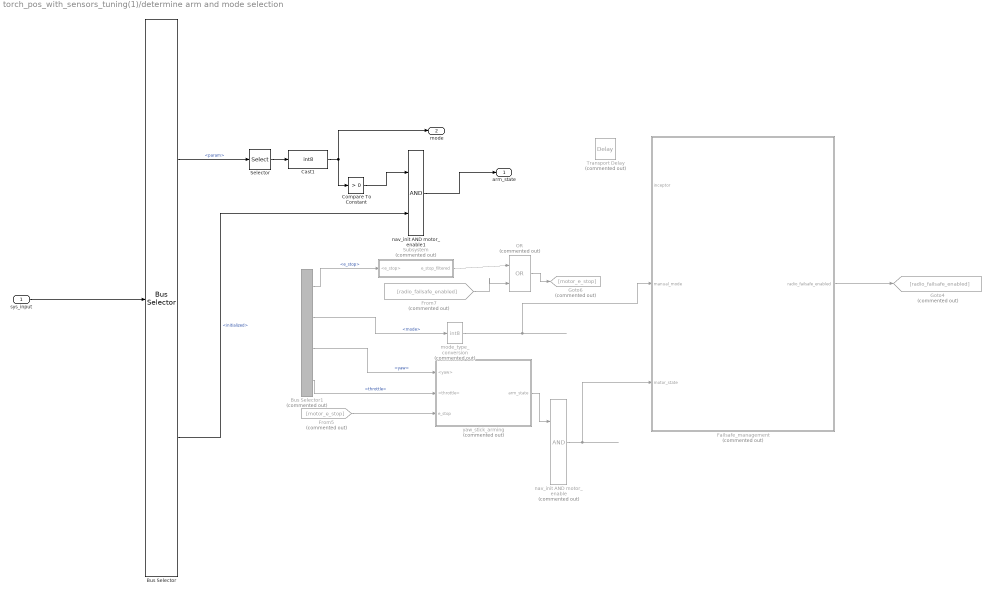
== system torch_pos_with_sensors_tuning(1)/determine arm and mode selection ==
  sys_input : Inport
  Bus Selector : BusSelector  OutputSignals=Telemetry Data.param,StateEstData.bfs_ins.initialized
  Bus Selector1 : BusSelector  Commented=on  OutputSignals=e_stop,mode,yaw,throttle
  Cast1 : DataTypeConversion  OutDataTypeStr=int8  SaturateOnIntegerOverflow=off  RndMeth=Floor
  Compare To Constant : simulink/Logic and Bit Operations/Compare To Constant  relop=>  const=0  OutDataTypeStr=boolean
  Failsafe_management : Subsystem  Commented=on
  From5 : From  Commented=on  GotoTag=motor_e_stop
  From7 : From  Commented=on  GotoTag=radio_failsafe_enabled
  Goto4 : Goto  Commented=on  GotoTag=radio_failsafe_enabled
  Goto6 : Goto  Commented=on  GotoTag=motor_e_stop
  OR : Logic  Commented=on  Operator=OR  IconShape=distinctive  AllPortsSameDT=off  OutDataTypeStr=boolean
  Selector : Selector  IndexMode=Zero-based  InputPortWidth=24  IndexOptions=Index vector (dialog)  Indices=0  OutputSizes=1
  Subsystem : Subsystem  Commented=on
  Transport Delay : TransportDelay  Commented=on
  mode_type_conversion : DataTypeConversion  Commented=on  OutDataTypeStr=int8  RndMeth=Nearest  SaturateOnIntegerOverflow=off
  nav_init AND motor_enable : Logic  Commented=on  IconShape=distinctive  AllPortsSameDT=off  OutDataTypeStr=boolean
  nav_init AND motor_enable1 : Logic  IconShape=distinctive  AllPortsSameDT=off  OutDataTypeStr=boolean
  yaw_stick_arming : Subsystem  Commented=on
  arm_state : Outport
  mode : Outport  Port=2
  wires:
  Selector/1 -> Cast1/1
  Bus Selector/1 -> Selector/1  "<param>"
  Bus Selector1/1 -> Subsystem/1(<e_stop>)  "<e_stop>"
  Cast1/1 -> Compare To Constant/1, mode/1
  OR/1 -> Goto6/1
  Bus Selector/2 -> nav_init AND motor_enable1/2  "<initialized>"
  nav_init AND motor_enable1/1 -> arm_state/1
  Compare To Constant/1 -> nav_init AND motor_enable1/1
  Subsystem/1(e_stop_filtered) -> OR/1
  Bus Selector1/4 -> yaw_stick_arming/2(<throttle>)  "<throttle>"
  From5/1 -> yaw_stick_arming/3(e_stop)
  Bus Selector1/3 -> yaw_stick_arming/1(<yaw>)  "<yaw>"
  yaw_stick_arming/1(arm_state) -> nav_init AND motor_enable/1
  nav_init AND motor_enable/1 -> Failsafe_management/3(motor_state)
  mode_type_conversion/1 -> Failsafe_management/2(manual_mode)
  Bus Selector1/2 -> mode_type_conversion/1  "<mode>"
  sys_input/1 -> Bus Selector/1
  Failsafe_management/1(radio_failsafe_enabled) -> Goto4/1
  From7/1 -> OR/2

== system torch_pos_with_sensors_tuning(1)/emergency_stop_system1 ==
  input_signal : Inport
  arm : Inport  Port=2
  Constant : Constant  Value=[0,0,0,0,0,0,0,0]  OutDataTypeStr=single
  emergency_switch : Switch  Criteria=u2 > Threshold  Threshold=0.5  SaturateOnIntegerOverflow=off  InputSameDT=off
  pwm_cmd : Outport
  wires:
  emergency_switch/1 -> pwm_cmd/1
  arm/1 -> emergency_switch/2
  input_signal/1 -> emergency_switch/1
  Constant/1 -> emergency_switch/3

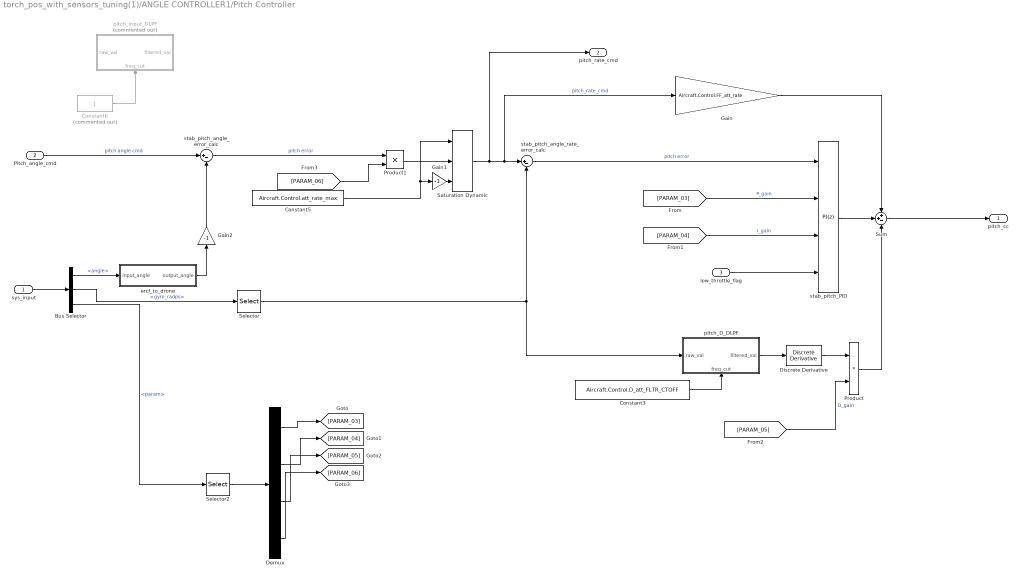
== system torch_pos_with_sensors_tuning(1)/ANGLE CONTROLLER1/Pitch Controller ==
  sys_input : Inport
  Pitch_angle_cmd : Inport  Port=2
  low_throttle_flag : Inport  Port=3
  Bus Selector : BusSelector  OutputSignals=Sensor Data.ercf.angle,StateEstData.bfs_ins.gyro_radps,Telemetry Data.param
  Constant3 : Constant  Value=Aircraft.Control.D_att_FLTR_CTOFF  OutDataTypeStr=single
  Constant5 : Constant  Value=Aircraft.Control.att_rate_max  OutDataTypeStr=single
  Constant6 : Constant  Commented=on  OutDataTypeStr=single
  Demux : Demux
  Discrete Derivative : simulink/Discrete/Discrete Derivative  gainval=1.0  ICPrevScaledInput=0.0  OutMin=[]  OutMax=[]  OutDataType=fixdt(1, 16)  OutScaling=2^-10  DoSatur=off
  Gain : Gain  Gain=Aircraft.Control.FF_att_rate
  Gain1 : Gain  Gain=-1
  Gain2 : Gain  Gain=-1
  Product : Product
  Product1 : Product
  Saturation Dynamic : simulink/Discontinuities/Saturation Dynamic  OutMin=[]  OutMax=[]  OutDataTypeStr=Inherit: Same as second input  OutDataType=fixdt(1, 16)  OutScaling=2^-10  DoSatur=off
  Selector : Selector  IndexMode=Zero-based  InputPortWidth=3  IndexOptions=Index vector (dialog)  Indices=1  OutputSizes=1
  Selector2 : Selector  IndexMode=Zero-based  InputPortWidth=24  IndexOptions=Index vector (dialog)  Indices=[3 4 5 6]  OutputSizes=1
  Sum : Sum  Inputs=++-
  ercf_to_drone : MATLAB Function  TreatAsAtomicUnit=on
  pitch_D_DLPF : Subsystem
      settings: PortSchema="{\"entries\":[{\"content\":{\"sides\":[{\"content\":{\"connectorIds\":[\"In1\"]},\"type\":\"ConnectorPlacement.EquallySpacedRectSide\",\"uuid\":\"20236834-aeb3-4c5b-bb2e-f84447e752b5\"},{\"content\":{\"connectorIds\":[\"Out1\"],\"side\":\"RIGHT\"},\"type\":\"ConnectorPlacement.EquallySpacedRectSide\",\"uuid\":\"d668f9a1-a3df-4207-8bf1-99fb838e59b2\"},{\"content\":{\"connectorIds\":[],\"side\":\"TOP\"},\"type\":\"ConnectorPlacement.EquallySpacedRectSide\",\"uuid\":\"66cceb06-f4bc-4278-b965-2427292e46df\"},{\"content\":{\"connectorIds\":[\"In2\"],\"side\":\"BOTTOM\"},\"type\":\"ConnectorPlacement.EquallySpacedRectSide\",\"uuid\":\"8fdaac6a-cb03-4bd4-87bb-7bafd10bc297\"}]},\"type\":\"ConnectorPlacement.EquallySpacedConnector\",\"uuid\":\"3dc29a9a-e794-478d-b7df-452e6c2d3f66\"}],\"packageUris\":[\"http://schema.mathworks.com/mf0/Connector/R2020b\"],\"version\":\"1.0\"}"
  pitch_input_DLPF : Subsystem  Commented=on
      settings: PortSchema="{\"entries\":[{\"content\":{\"sides\":[{\"content\":{\"connectorIds\":[\"In1\"]},\"type\":\"ConnectorPlacement.EquallySpacedRectSide\",\"uuid\":\"20236834-aeb3-4c5b-bb2e-f84447e752b5\"},{\"content\":{\"connectorIds\":[\"Out1\"],\"side\":\"RIGHT\"},\"type\":\"ConnectorPlacement.EquallySpacedRectSide\",\"uuid\":\"d668f9a1-a3df-4207-8bf1-99fb838e59b2\"},{\"content\":{\"connectorIds\":[],\"side\":\"TOP\"},\"type\":\"ConnectorPlacement.EquallySpacedRectSide\",\"uuid\":\"66cceb06-f4bc-4278-b965-2427292e46df\"},{\"content\":{\"connectorIds\":[\"In2\"],\"side\":\"BOTTOM\"},\"type\":\"ConnectorPlacement.EquallySpacedRectSide\",\"uuid\":\"8fdaac6a-cb03-4bd4-87bb-7bafd10bc297\"}]},\"type\":\"ConnectorPlacement.EquallySpacedConnector\",\"uuid\":\"3dc29a9a-e794-478d-b7df-452e6c2d3f66\"}],\"packageUris\":[\"http://schema.mathworks.com/mf0/Connector/R2020b\"],\"version\":\"1.0\"}"
  stab_pitch_PID : slpidlib/PID Controller  Controller=PI  Form=Parallel  TimeDomain=Discrete-time  UseExternalTs=off  SampleTime=framePeriod_s  IntegratorMethod=Forward Euler  FilterMethod=Forward Euler  ControllerParametersSource=external  P=0.335  I=0.005  UseKiTs=off  D=0  UseExternalDerivativeSource=off  N=100  UseFilter=off  TunerSelectOption=Transfer Function Based (PID Tuner App)  InitialConditionSource=internal  InitialConditionForIntegrator=0  InitialConditionForFilter=0  DifferentiatorICPrevScaledInput=0  ExternalReset=either  TrackingMode=off  Kt=1  LimitOutput=on  SatLimitsSource=internal  UpperSaturationLimit=1  LowerSaturationLimit=-1  LinearizeAsGain=on  AntiWindupMode=clamping  Kb=1  LimitIntegrator=off  UpperIntegratorSaturationLimit=inf  LowerIntegratorSaturationLimit=-inf  POutMin=[]  POutMax=[]  IOutMin=[]  IOutMax=[]  DOutMin=[]  DOutMax=[]  NOutMin=[]  NOutMax=[]  SumOutMin=[]  SumOutMax=[]  SaturationOutMin=[]  SaturationOutMax=[]  PParamMin=[]  PParamMax=[]  IParamMin=[]  IParamMax=[]  DParamMin=[]  DParamMax=[]  NParamMin=[]  NParamMax=[]  KbParamMin=[]  KbParamMax=[]  KtParamMin=[]  KtParamMax=[]  KbOutMin=[]  KbOutMax=[]  KtOutMin=[]  KtOutMax=[]  IntegratorOutMin=[]  IntegratorOutMax=[]  FilterOutMin=[]  FilterOutMax=[]  SumI1OutMin=[]  SumI1OutMax=[]  SumI2OutMin=[]  SumI2OutMax=[]  SumI3OutMin=[]  SumI3OutMax=[]  SumI4OutMin=[]  SumI4OutMax=[]  SumDOutMin=[]  SumDOutMax=[]  DifferentiatorOutMin=[]  DifferentiatorOutMax=[]  FilterDiffOutCoefMin=[]  FilterDiffOutCoefMax=[]  ReciprocalOutMin=[]  ReciprocalOutMax=[]  SumDenOutMin=[]  SumDenOutMax=[]  SumNumOutMin=[]  SumNumOutMax=[]  DivideOutMin=[]  DivideOutMax=[]  UdiffTsProdOutMin=[]  UdiffTsProdOutMax=[]  NTsProdOutMin=[]  NTsProdOutMax=[]  UintegralTsProdOutMin=[]  UintegralTsProdOutMax=[]  UngainTsProdOutMin=[]  UngainTsProdOutMax=[]  ClampingZeroOutDataTypeStr=Inherit: Inherit via back propagation  ClampingZeroOutMin=[]  ClampingZeroOutMax=[]  FilterDenConstantOutDataTypeStr=Inherit: Inherit via back propagation  FilterDenConstantOutMin=[]  FilterDenConstantOutMax=[]  PCopyOutDataTypeStr=Inherit: Inherit via back propagation  PCopyOutMin=[]  PCopyOutMax=[]  NCopyOutDataTypeStr=Inherit: Inherit via back propagation  NCopyOutMin=[]  NCopyOutMax=[]  IntegratorContinuousStateAttributes=''  IntegratorStateMustResolveToSignalObject=off  IntegratorRTWStateStorageClass=Auto  FilterContinuousStateAttributes=''  FilterStateMustResolveToSignalObject=off  FilterRTWStateStorageClass=Auto  ParallelPVariant=ExternalParameters  IdealPVariant=Disabled  IVariant=ExternalParameters  DVariant=Disabled  IntegratorVariant=Discrete  SatVariant=Enabled  AWVariant=DiscClampingParallel  PCopyVariant=Disabled  TRVariant=Disabled  FdbkBlocksVariant=Forward  IdealPFdbkVariant=Disabled  SatFdbkVariant=Disabled  DerivativeFilterVariant=Disabled  NVariant=Disabled  NCopyVariant=Disabled_SignalSpec  FilterICVariant=Disabled  IntegratorICVariant=InternalICs  ExternalResetVariant=ExternalReset  TRSumVariant=Passthrough  SumFdbkVariant=Disabled  SumVariant=Sum_PI  TsampFilterVariant=InternalTs  TsampNgainVariant=Passthrough  TsampIntegralVariant=Disabled_SignalSpec  ExternalSaturationOutDataTypeStr=Inherit: Same as second input  DerivativeSourceVariant=Disabled
  stab_pitch_angle_error_calc : Sum  Inputs=|+-
  stab_pitch_angle_rate_error_calc : Sum  Inputs=|+-
  pitch_cc : Outport
  pitch_rate_cmd : Outport  Port=2
  wires:
  sys_input/1 -> Bus Selector/1
  Bus Selector/1 -> ercf_to_drone/1(input_angle)  "<angle>"
  Sum/1 -> pitch_cc/1
  Bus Selector/2 -> Selector/1  "<gyro_radps>"
  [PARAM_03] -> stab_pitch_PID/2  "P_gain"
  [PARAM_04] -> stab_pitch_PID/3  "I_gain"
  [PARAM_05] -> Product/2  "D_gain"
  low_throttle_flag/1 -> stab_pitch_PID/4
  Selector/1 -> stab_pitch_angle_rate_error_calc/2, pitch_D_DLPF/1(raw_val)
  stab_pitch_angle_error_calc/1 -> Product1/1  "pitch error"
  [PARAM_06] -> Product1/2
  Gain1/1 -> Saturation Dynamic/3
  Product1/1 -> Saturation Dynamic/2
  Discrete Derivative/1 -> Product/1
  Constant5/1 -> Saturation Dynamic/1, Gain1/1
  Constant3/1 -> pitch_D_DLPF/2(freq_cut)
  pitch_D_DLPF/1(filtered_val) -> Discrete Derivative/1
  stab_pitch_angle_rate_error_calc/1 -> stab_pitch_PID/1  "pitch error"
  Saturation Dynamic/1 -> pitch_rate_cmd/1, Gain/1, stab_pitch_angle_rate_error_calc/1  "pitch_rate_cmd"
  Constant6/1 -> pitch_input_DLPF/2(freq_cut)
  Pitch_angle_cmd/1 -> stab_pitch_angle_error_calc/1  "pitch angle cmd"
  Gain/1 -> Sum/1
  stab_pitch_PID/1 -> Sum/2
  Product/1 -> Sum/3
  ercf_to_drone/1(output_angle) -> Gain2/1
  Gain2/1 -> stab_pitch_angle_error_calc/2
  Demux/1 -> [PARAM_03]
  Selector2/1 -> Demux/1
  Demux/3 -> [PARAM_05]
  Bus Selector/3 -> Selector2/1  "<param>"
  Demux/2 -> [PARAM_04]
  Demux/4 -> [PARAM_06]

== system torch_pos_with_sensors_tuning(1)/POS_HOLD CONTROLLER/Horizontal speed controller ==
  note: Assume small roll and pitch angles so translation in Earth frame can be rotated to body frame by rotating by heading only
  sys_input : Inport
  ve_x_cmd_mps : Inport  Port=2
  pos_hold_init : Inport  Port=3
  Bus Creator : BusCreator  Inputs=3
  Bus Selector : BusSelector  OutputSignals=Sensor Data.tfmini.range_cm,StateEstData.bfs_ins.ned_vel_mps
  Bus Selector1 : BusSelector  OutputSignals=ve_x_cmd,ve_x
  Cast To Single : DataTypeConversion  OutDataTypeStr=single  SaturateOnIntegerOverflow=off  RndMeth=Floor
  Gain : Gain  Gain=0.01
  Selector : Selector  InputPortWidth=3  IndexOptions=Index vector (dialog)  Indices=1  OutputSizes=1
  Subsystem : Subsystem
  zero_vel_handling : Subsystem
  acc_x_cmd : Outport
  Output : Outport  Port=2
  target : Outport  Port=3
  wires:
  Subsystem/1(acc_x_cmd) -> acc_x_cmd/1  "acc_x_cmd"
  sys_input/1 -> Bus Selector/1
  Bus Selector/2 -> Selector/1  "<ned_vel_mps>"
  pos_hold_init/1 -> [pos_hold_init]
  [pos_hold_init] -> Subsystem/3(pos_hold_init)
  Subsystem/2(Output) -> Bus Selector1/1
  Bus Selector1/1 -> Bus Creator/1  "<ve_x_cmd>"
  Bus Selector1/2 -> Bus Creator/2  "<ve_x>"
  Bus Creator/1 -> Output/1
  Bus Selector/1 -> Gain/1  "<range_cm>"
  ve_x_cmd_mps/1 -> zero_vel_handling/1(ve_x cmd)
  Gain/1 -> Cast To Single/1  "pos_e_xy"
  [pos_hold_init] -> zero_vel_handling/3(pos_hold_init)
  zero_vel_handling/1(v_cmd) -> Subsystem/1(ve_x cmd)
  zero_vel_handling/2(Output) -> Bus Creator/3  "tar_x"
  Selector/1 -> Subsystem/2(ve_x)  "ve_xy"
  zero_vel_handling/3(tar_get) -> target/1
  Cast To Single/1 -> zero_vel_handling/2(pos_e_feedback)
